simulink model "Model_2DoF_m1_14b"  (R2014b)
settings: Solver=ode45  StartTime=0.0  StopTime=10  MaxStep=0.2  RelTol=1e-3
undefined symbols (not defined in the file or in its folder): in, param
settings Model: Creator=Zer0  LastModifiedBy=Arek

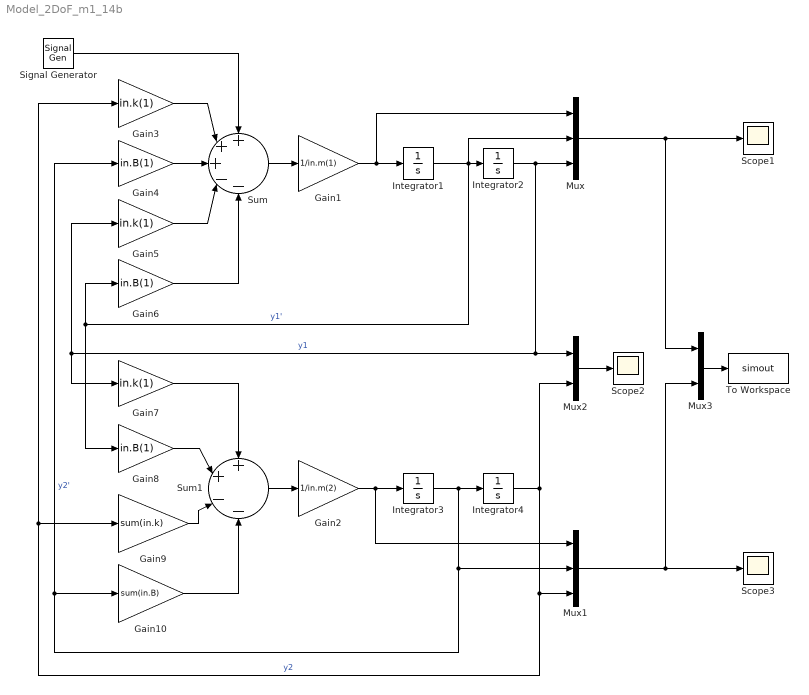
== system Model_2DoF_m1_14b ==
  Gain1 : Gain  Gain=1/in.m(1)
  Gain10 : Gain  Gain=sum(in.B)
  Gain2 : Gain  Gain=1/in.m(2)
  Gain3 : Gain  Gain=in.k(1)
  Gain4 : Gain  Gain=in.B(1)
  Gain5 : Gain  Gain=in.k(1)
  Gain6 : Gain  Gain=in.B(1)
  Gain7 : Gain  Gain=in.k(1)
  Gain8 : Gain  Gain=in.B(1)
  Gain9 : Gain  Gain=sum(in.k)
  Integrator1 : Integrator  InitialCondition=param.ic(2)
  Integrator2 : Integrator  InitialCondition=param.ic(1)
  Integrator3 : Integrator  InitialCondition=param.ic(4)
  Integrator4 : Integrator  InitialCondition=param.ic(3)
  Mux : Mux  Inputs=3
  Mux1 : Mux  Inputs=3
  Mux2 : Mux  Inputs=2
  Mux3 : Mux  Inputs=2
  Scope1 : Scope
  Scope2 : Scope
      settings: YMin=-1  YMax=1  SaveName=ScopeData2
  Scope3 : Scope
  Signal Generator : SignalGenerator  Amplitude=in.F
  Sum : Sum  Inputs=+|+|+|-|-
  Sum1 : Sum  Inputs=+|+|-|-
  To Workspace : ToWorkspace  VariableName=simout  SaveFormat=Timeseries  SampleTime=-1
  wires:
  Integrator3/1 -> Mux1/2, Gain4/1, Gain10/1, Integrator4/1  "y2'"
  Integrator1/1 -> Mux/2, Integrator2/1, Gain8/1, Gain6/1  "y1'"
  Mux3/1 -> To Workspace/1
  Mux2/1 -> Scope2/1
  Gain6/1 -> Sum/5
  Gain4/1 -> Sum/3
  Gain3/1 -> Sum/2
  Gain5/1 -> Sum/4
  Gain7/1 -> Sum1/1
  Gain8/1 -> Sum1/2
  Integrator2/1 -> Mux/3, Mux2/1, Gain5/1, Gain7/1  "y1"
  Integrator4/1 -> Mux1/3, Gain3/1, Gain9/1, Mux2/2  "y2"
  Mux1/1 -> Scope3/1, Mux3/2
  Mux/1 -> Scope1/1, Mux3/1
  Gain1/1 -> Mux/1, Integrator1/1
  Sum/1 -> Gain1/1
  Gain2/1 -> Integrator3/1, Mux1/1
  Sum1/1 -> Gain2/1
  Gain9/1 -> Sum1/3
  Gain10/1 -> Sum1/4
  Signal Generator/1 -> Sum/1
